simulink model "inlab_task"  (R2015a)
settings: Solver=ode45  StartTime=0.0  StopTime=50  RelTol=1e-3
libraries: powerlib x4
settings Model: Creator=Syed_Sharjeel  LastModifiedBy=Syed_Sharjeel

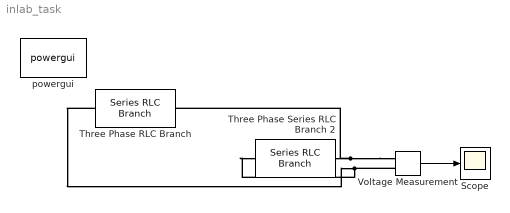
== system inlab_task ==
  " Three Phase Series RLC Branch 2" : powerlib/Elements/Series RLC Branch  LConnTagsString=__new0  RConnTagsString=__new0  BranchType=C  Resistance=3  Inductance=1  SetiL0=off  InitialCurrent=0  Capacitance=1.5  Setx0=on  InitialVoltage=5  Measurements=None
  Scope : Scope
      settings: TimeRange=10  YMin=4  YMax=6
  "Three Phase RLC Branch " : powerlib/Elements/Series RLC Branch  LConnTagsString=__new0  RConnTagsString=__new0  BranchType=RL  Resistance=3  Inductance=1  SetiL0=off  InitialCurrent=0  Capacitance=1.5  Setx0=off  InitialVoltage=0  Measurements=None
  Voltage Measurement : powerlib/Measurements/Voltage Measurement  PhasorSimulation=off  OutputType=Complex  PSBequivalent=0
  powergui : powerlib/powergui  Priority=1  SimulationMode=Continuous  SolverType=Tustin/Backward Euler (TBE)  SampleTime=50e-6  frequency=60  SPID=off  DisableSnubberDevices=off  DisableRonSwitches=off  DisableVfSwitches=off  SwTol=0  DisplayEquations=off  Interpol=off  methode=off  Ts=100  FunctionMessages=off  echomessages=off  HookPort=off  EnableUseOfTLC=off  x0status=blocks  frequencyindice=60  Pbase=100e6  ErrMax=1e-4  Iterations=50  UnitsV=kV  UnitsW=MW  buscounter=0  RestoreLinks=warning  ResistiveCurrentMeasurement=off  Frange=[0:2:500]  Ylog=off  Xlog=on  ShowGrid=off  save=off  variable=ZData  structure=0  ZoomFFT=off  StartTime=0.0  cycles=1  DisplayStyle=1  fundamental=60  FreqAxis=off  MaxFrequency=1000  frequencyindicesteady=1  RmsSteady=1  display=off
  wires:
  Voltage Measurement/1 -> Scope/1
  connections:
  " Three Phase Series RLC Branch 2"/RConn1 -- "Three Phase RLC Branch "/LConn1 -- Voltage Measurement/LConn2
  Voltage Measurement/LConn1 -- "Three Phase RLC Branch "/RConn1 -- " Three Phase Series RLC Branch 2"/LConn1
